simulink model "Sim2"  (R2024b)
settings: Solver=VariableStepAuto  StartTime=0.0  StopTime=25  RelTol=1e-3
values from neighbouring files (symbols this model uses):
  g = 9.8    [code.m]
  jw = 0.01    [code.m]
  K = 1000    [code.m]
  mv = 1400    [code.m]
  roadType = 4    [code.m]
  rw = 0.32    [code.m]
  T = 0.05    [code.m]
  v0 = 33.33    [code.m]
  Vmin = 1.5    [code.m]
settings Model: Creator=amira  LastModifiedBy=Ali
settings DataIOCC: ReturnWorkspaceOutputs=off
settings OptimizationCC: ReuseModelBlockBuffer=off
settings RTWCC: GPUComputeCapability=3.5

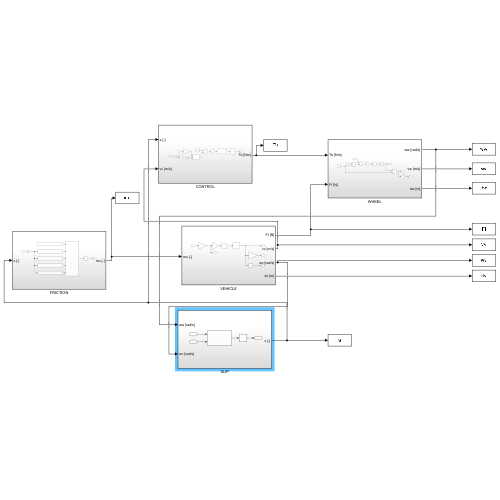
[thumbnail: Simulink's stored preview of the top-level diagram]
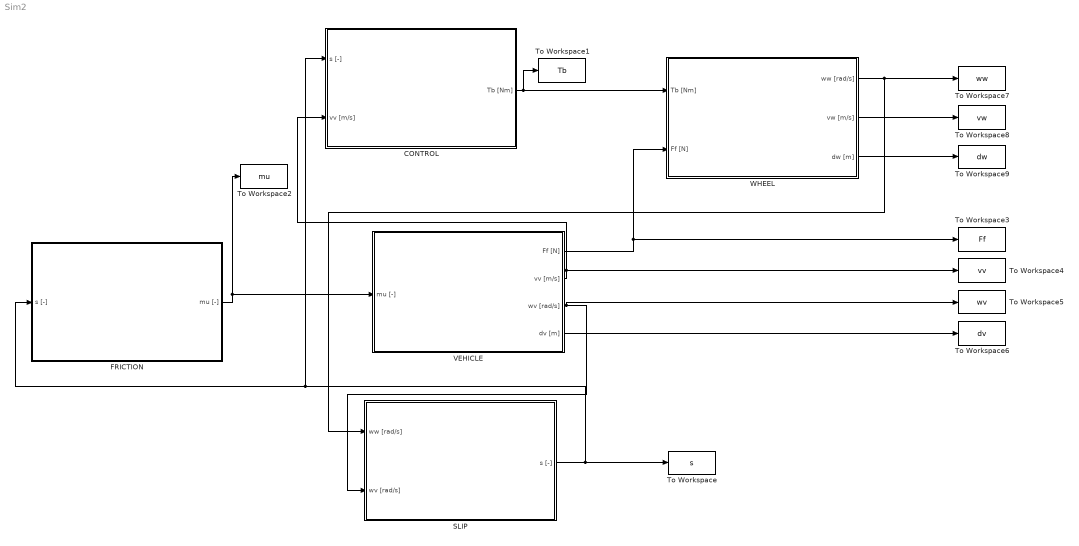
== system Sim2 ==
  CONTROL : Subsystem
  FRICTION : Subsystem
  SLIP : Subsystem
  To Workspace : ToWorkspace  VariableName=s  SaveFormat=Timeseries  SampleTime=-1
  To Workspace1 : ToWorkspace  VariableName=Tb  SaveFormat=Timeseries  SampleTime=-1
  To Workspace2 : ToWorkspace  VariableName=mu  SaveFormat=Timeseries  SampleTime=-1
  To Workspace3 : ToWorkspace  VariableName=Ff  SaveFormat=Timeseries  SampleTime=-1
  To Workspace4 : ToWorkspace  VariableName=vv  SaveFormat=Timeseries  SampleTime=-1
  To Workspace5 : ToWorkspace  VariableName=wv  SaveFormat=Timeseries  SampleTime=-1
  To Workspace6 : ToWorkspace  VariableName=dv  SaveFormat=Timeseries  SampleTime=-1
  To Workspace7 : ToWorkspace  VariableName=ww  SaveFormat=Timeseries  SampleTime=-1
  To Workspace8 : ToWorkspace  VariableName=vw  SaveFormat=Timeseries  SampleTime=-1
  To Workspace9 : ToWorkspace  VariableName=dw  SaveFormat=Timeseries  SampleTime=-1
  VEHICLE : Subsystem
  WHEEL : Subsystem
  wires:
  VEHICLE/4(dv [m]) -> To Workspace6/1
  WHEEL/1(ww [rad/s]) -> To Workspace7/1, SLIP/1(ww [rad/s])
  VEHICLE/3(wv [rad/s]) -> SLIP/2(wv [rad/s]), To Workspace5/1
  WHEEL/2(vw [m/s]) -> To Workspace8/1
  VEHICLE/2(vv [m/s]) -> CONTROL/2(vv [m/s]), To Workspace4/1
  WHEEL/3(dw [m]) -> To Workspace9/1
  VEHICLE/1(Ff [N]) -> WHEEL/2(Ff [N]), To Workspace3/1
  SLIP/1(s [-]) -> CONTROL/1(s [-]), FRICTION/1(s [-]), To Workspace/1
  FRICTION/1(mu [-]) -> To Workspace2/1, VEHICLE/1(mu [-])
  CONTROL/1(Tb [Nm]) -> WHEEL/1(Tb [Nm]), To Workspace1/1

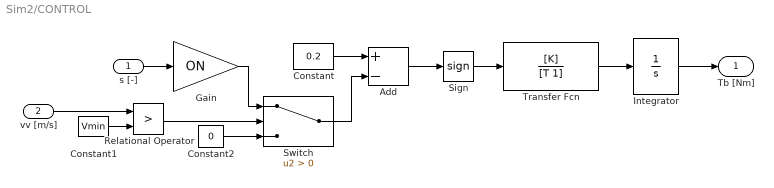
== system Sim2/CONTROL ==
  s [-] : Inport
  vv [m/s] : Inport  Port=2
  Add : Sum  Inputs=+-
  Constant : Constant  Value=0.2
  Constant1 : Constant  Value=Vmin
  Constant2 : Constant  Value=0
  Gain : Gain  Gain=ON
  Integrator : Integrator  LimitOutput=on  UpperSaturationLimit=2000  LowerSaturationLimit=0
  Relational Operator : RelationalOperator  Operator=>  OutDataTypeStr=boolean  RndMeth=Simplest  InputSameDT=off
  Sign : Signum
  Switch : Switch  Criteria=u2 > Threshold  SaturateOnIntegerOverflow=off  InputSameDT=off
  Transfer Fcn : TransferFcn  Numerator=[K]  Denominator=[T 1]
  Tb [Nm] : Outport  VectorParamsAs1DForOutWhenUnconnected=off
  wires:
  Add/1 -> Sign/1
  Constant2/1 -> Switch/3
  Transfer Fcn/1 -> Integrator/1
  Integrator/1 -> Tb [Nm]/1
  Relational Operator/1 -> Switch/2
  vv [m/s]/1 -> Relational Operator/1
  s [-]/1 -> Gain/1
  Constant1/1 -> Relational Operator/2
  Constant/1 -> Add/1
  Sign/1 -> Transfer Fcn/1
  Switch/1 -> Add/2
  Gain/1 -> Switch/1

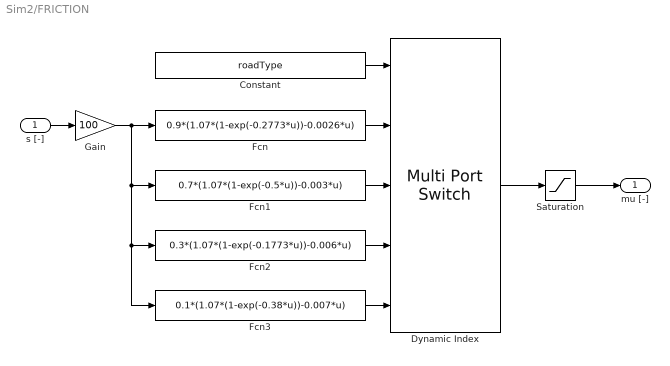
== system Sim2/FRICTION ==
  s [-] : Inport
  Constant : Constant  Value=roadType
  Dynamic Index : MultiPortSwitch  Inputs=4  SaturateOnIntegerOverflow=off  InputSameDT=off
  Fcn : Fcn  Expr=0.9*(1.07*(1-exp(-0.2773*u))-0.0026*u)
  Fcn1 : Fcn  Expr=0.7*(1.07*(1-exp(-0.5*u))-0.003*u)
  Fcn2 : Fcn  Expr=0.3*(1.07*(1-exp(-0.1773*u))-0.006*u)
  Fcn3 : Fcn  Expr=0.1*(1.07*(1-exp(-0.38*u))-0.007*u)
  Gain : Gain  Gain=100
  Saturation : Saturate  UpperLimit=1  LowerLimit=0
  mu [-] : Outport  VectorParamsAs1DForOutWhenUnconnected=off
  wires:
  Fcn3/1 -> Dynamic Index/5
  Saturation/1 -> mu [-]/1
  Fcn/1 -> Dynamic Index/2
  Fcn2/1 -> Dynamic Index/4
  Gain/1 -> Fcn3/1, Fcn2/1, Fcn1/1, Fcn/1
  s [-]/1 -> Gain/1
  Fcn1/1 -> Dynamic Index/3
  Constant/1 -> Dynamic Index/1
  Dynamic Index/1 -> Saturation/1

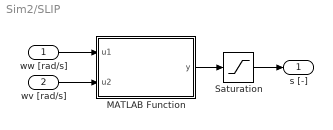
== system Sim2/SLIP ==
  ww [rad/s] : Inport
  wv [rad/s] : Inport  Port=2
  MATLAB Function : MATLAB Function  TreatAsAtomicUnit=on
  Saturation : Saturate  UpperLimit=1  LowerLimit=0
  s [-] : Outport  VectorParamsAs1DForOutWhenUnconnected=off
  wires:
  wv [rad/s]/1 -> MATLAB Function/2(u2)
  ww [rad/s]/1 -> MATLAB Function/1(u1)
  Saturation/1 -> s [-]/1
  MATLAB Function/1(y) -> Saturation/1

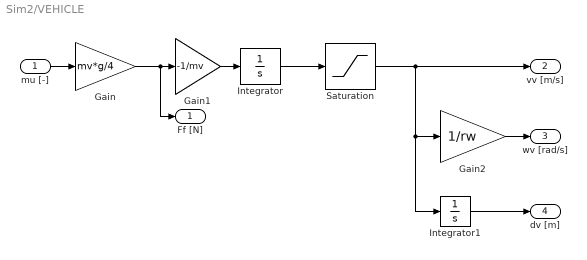
== system Sim2/VEHICLE ==
  mu [-] : Inport
  Gain : Gain  Gain=mv*g/4
  Gain1 : Gain  Gain=-1/mv
  Gain2 : Gain  Gain=1/rw
  Integrator : Integrator  InitialCondition=v0
  Integrator1 : Integrator
  Saturation : Saturate  UpperLimit=1000  LowerLimit=0.001
  Ff [N] : Outport  VectorParamsAs1DForOutWhenUnconnected=off
  vv [m/s] : Outport  Port=2  VectorParamsAs1DForOutWhenUnconnected=off
  wv [rad/s] : Outport  Port=3  VectorParamsAs1DForOutWhenUnconnected=off
  dv [m] : Outport  Port=4  VectorParamsAs1DForOutWhenUnconnected=off
  wires:
  Gain2/1 -> wv [rad/s]/1
  Saturation/1 -> vv [m/s]/1, Integrator1/1, Gain2/1
  Gain/1 -> Ff [N]/1, Gain1/1
  Integrator1/1 -> dv [m]/1
  mu [-]/1 -> Gain/1
  Integrator/1 -> Saturation/1
  Gain1/1 -> Integrator/1

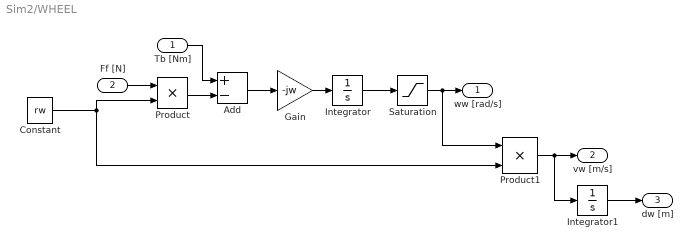
== system Sim2/WHEEL ==
  Tb [Nm] : Inport
  Ff [N] : Inport  Port=2
  Add : Sum  Inputs=+-
  Constant : Constant  Value=rw
  Gain : Gain  Gain=-jw
  Integrator : Integrator  InitialCondition=v0/rw
  Integrator1 : Integrator
  Product : Product
  Product1 : Product
  Saturation : Saturate  UpperLimit=1000  LowerLimit=0
  ww [rad/s] : Outport  VectorParamsAs1DForOutWhenUnconnected=off
  vw [m/s] : Outport  Port=2  VectorParamsAs1DForOutWhenUnconnected=off
  dw [m] : Outport  Port=3  VectorParamsAs1DForOutWhenUnconnected=off
  wires:
  Product/1 -> Add/2
  Saturation/1 -> Product1/1, ww [rad/s]/1
  Gain/1 -> Integrator/1
  Product1/1 -> vw [m/s]/1, Integrator1/1
  Constant/1 -> Product/2, Product1/2
  Tb [Nm]/1 -> Add/1
  Integrator/1 -> Saturation/1
  Integrator1/1 -> dw [m]/1
  Ff [N]/1 -> Product/1
  Add/1 -> Gain/1

== matlab function Sim2/SLIP/MATLAB Function ==
  data: u1 input; y output; u2 input
function y = fcn(u1,u2)
y = 1 - (u1/(u2+(u2==0)*eps))
end
